simulink model "P2Simulink"  (R2023b)
settings: Solver=VariableStepAuto  StartTime=0.0  StopTime=100  FixedStep=1  RelTol=1e-3
undefined symbols (not defined in the file or in its folder): DiscIntNeverNeededParam, K, kw, LA, R, tau, Ts, x, y
settings Model: PauseTimes=100  Creator=rpl  LastModifiedBy=rpl

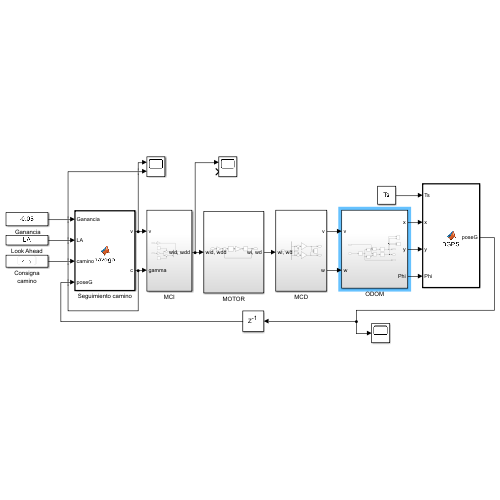
[thumbnail: Simulink's stored preview of the top-level diagram]
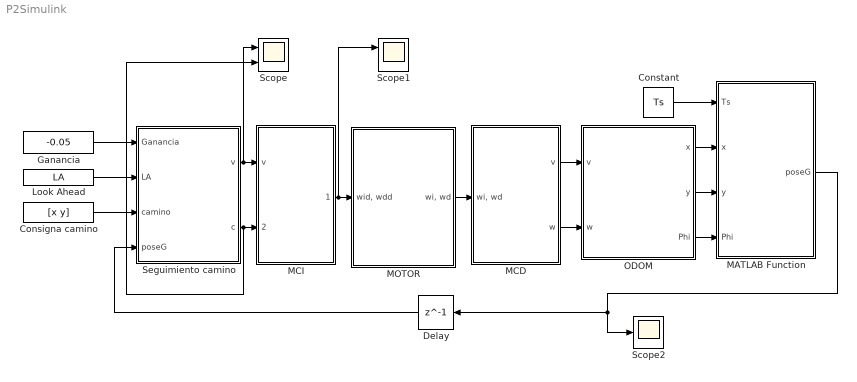
== system P2Simulink ==
  " Ganancia" : Constant  Value=-0.05
  Consigna camino : Constant  Value=[x y]  SampleTime=Ts
  Constant : Constant  Value=Ts
  Delay : Delay  DelayLength=1  InitialCondition=[0; 0; 0]
  Look Ahead : Constant  Value=LA
  MATLAB Function : MATLAB Function  TreatAsAtomicUnit=on
  MCD : Subsystem
  MCI : Subsystem
  MOTOR : Subsystem
  ODOM : Subsystem
  Scope : Scope  NumInputPorts=2
  Scope1 : Scope  NumInputPorts=2
  Scope2 : Scope
  Seguimiento camino : MATLAB Function  TreatAsAtomicUnit=on
  wires:
  MOTOR/1("wi, wd") -> MCD/1("wi, wd")
  Consigna camino/1 -> Seguimiento camino/3(camino)
  MCD/1(v) -> ODOM/1(v)
  MCD/2(w) -> ODOM/2(w)
  MATLAB Function/1(poseG) -> Scope2/1, Delay/1
  MCI/1("wid, wdd") -> Scope1/1, MOTOR/1("wid, wdd")
  Seguimiento camino/1(v) -> Scope/1, MCI/1(v)
  Seguimiento camino/2(c) -> Scope/2, MCI/2(gamma)
  " Ganancia"/1 -> Seguimiento camino/1(Ganancia)
  Constant/1 -> MATLAB Function/1(Ts)
  Look Ahead/1 -> Seguimiento camino/2(LA)
  Delay/1 -> Seguimiento camino/4(poseG)
  ODOM/1(x) -> MATLAB Function/2(x)
  ODOM/2(y) -> MATLAB Function/3(y)
  ODOM/3(Phi) -> MATLAB Function/4(Phi)

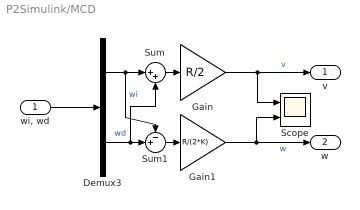
== system P2Simulink/MCD ==
  "wi, wd" : Inport
  Demux3 : Demux  Outputs=2
  Gain : Gain  Gain=R/2
  Gain1 : Gain  Gain=R/(2*K)
  Scope : Scope  NumInputPorts=2
  Sum : Sum  Inputs=|++
  Sum1 : Sum  Inputs=-+|
  v : Outport
  w : Outport  Port=2
  wires:
  Sum/1 -> Gain/1
  Gain/1 -> Scope/1, v/1  "v"
  Demux3/2 -> Sum/2, Sum1/2  "wd"
  Demux3/1 -> Sum1/1, Sum/1  "wi"
  Sum1/1 -> Gain1/1
  Gain1/1 -> Scope/2, w/1  "w"
  "wi, wd"/1 -> Demux3/1

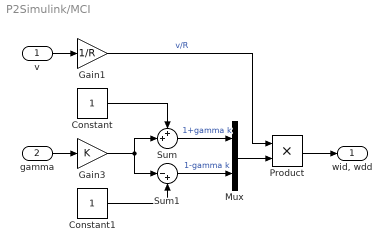
== system P2Simulink/MCI ==
  v : Inport
  gamma : Inport  Port=2
  Constant : Constant
  Constant1 : Constant
  Gain1 : Gain  Gain=1/R
  Gain3 : Gain  Gain=K
  Mux : Mux  Inputs=2
  Product : Product
  Sum : Sum  Inputs=++|
  Sum1 : Sum  Inputs=|-+
  "wid, wdd" : Outport
  wires:
  v/1 -> Gain1/1
  Sum/1 -> Mux/1  "1+gamma k"
  Mux/1 -> Product/2
  Sum1/1 -> Mux/2  "1-gamma k"
  gamma/1 -> Gain3/1
  Gain1/1 -> Product/1  "v/R"
  Product/1 -> "wid, wdd"/1
  Constant/1 -> Sum/1
  Gain3/1 -> Sum1/1, Sum/2
  Constant1/1 -> Sum1/2

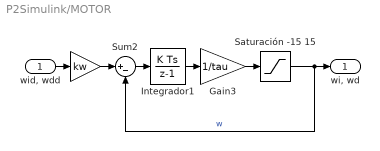
== system P2Simulink/MOTOR ==
  "wid, wdd" : Inport
  " " : Gain  Gain=kw
  Gain3 : Gain  Gain=1/tau
  Integrador1 : DiscreteIntegrator  SampleTime=-1  ICPrevOutput=DiscIntNeverNeededParam  ICPrevScaledInput=DiscIntNeverNeededParam
  Saturación -15 15 : Saturate  UpperLimit=15  LowerLimit=-15
  Sum2 : Sum  Inputs=|+-
  "wi, wd" : Outport
  wires:
  Gain3/1 -> Saturación -15 15/1
  Integrador1/1 -> Gain3/1
  Sum2/1 -> Integrador1/1
  Saturación -15 15/1 -> Sum2/2, "wi, wd"/1  "w"
  "wid, wdd"/1 -> " "/1
  " "/1 -> Sum2/1

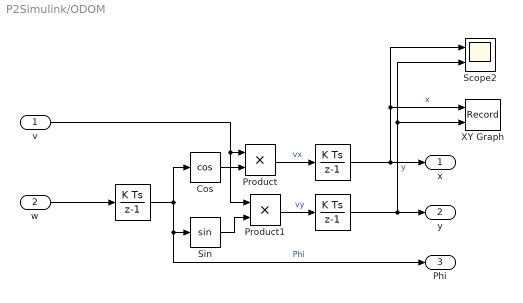
== system P2Simulink/ODOM ==
  v : Inport
  w : Inport  Port=2
  " " : DiscreteIntegrator  SampleTime=-1  ICPrevOutput=DiscIntNeverNeededParam  ICPrevScaledInput=DiscIntNeverNeededParam
  "  " : DiscreteIntegrator  SampleTime=-1  ICPrevOutput=DiscIntNeverNeededParam  ICPrevScaledInput=DiscIntNeverNeededParam
  "   " : DiscreteIntegrator  SampleTime=-1  ICPrevOutput=DiscIntNeverNeededParam  ICPrevScaledInput=DiscIntNeverNeededParam
  Cos : Trigonometry  Operator=cos
  Product : Product
  Product1 : Product
  Scope2 : Scope  NumInputPorts=2
  Sin : Trigonometry
  XY Graph : Record  FileSettingsInternal="{\"entries\":[{\"content\":{\"excelSettings\":{\"content\":{},\"type\":\"Streamout.ExcelSettings\"}},\"type\":\"Streamout.FileSettingStorage\",\"uuid\":\"\"}],\"packageUris\":[\"http:\\/\\/schema.mathworks.com\\/mf0\\/streamout_blocks\\/R2020a\"],\"version\":\"1.0\"}"  Layout=[1 1]  SignalsInternal="{\"entries\":[{\"content\":{\"signals\":[{\"content\":{\"blockPath\":[],\"dimensions\":[1],\"domain\":\"\",\"lineColor\":\"#a2142f\",\"plots\":[ 1 ],\"port\":1,\"sid\":[\"\"],\"signalID\":1,\"signalName\":\"x\"},\"type\":\"RecordBlkView.Signal\",\"uuid\":\"\"},{\"content\":{\"blockPath\":[],\"dimensions\":[1],\"domain\":\"\",\"lineColor\":\"#139fff\",\"plots\":[ 1 ],\"port\":2,\"sid\":[\"\"],\"signalID\":2,\"signalName\":\"y\"},\"type\":\"RecordBlkView.Signal\",\"uuid\":\"\"}]},\"type\":\"RecordBlkView.InputSignals\",\"uuid\":\"\"}],\"packageUris\":[\"http:\\/\\/schema.mathworks.com\\/mf0\\/streamout_blocks\\/R2020a\"],\"version\":\"1.0\"}"  VisualizationBindings="{\"xyplotplugin\":{\"info\":[{\"series\":[{\"bindingParametersList\":[{\"parameter\":\"X-Axis\",\"signalID\":1,\"signalName\":\"x\"},{\"parameter\":\"Y-Axis\",\"signalID\":2,\"signalName\":\"y\"}],\"seriesID\":0}],\"subplotID\":1}]}}"  CompatibilityTag=XY
  x : Outport
  y : Outport  Port=2
  Phi : Outport  Port=3
  wires:
  Cos/1 -> Product/2
  w/1 -> "   "/1
  "   "/1 -> Cos/1, Phi/1, Sin/1  "Phi"
  Product/1 -> "  "/1  "vx"
  Sin/1 -> Product1/2
  "  "/1 -> x/1, Scope2/1, XY Graph/1  "x"
  v/1 -> Product1/1, Product/1
  Product1/1 -> " "/1  "vy"
  " "/1 -> y/1, XY Graph/2, Scope2/2  "y"

== matlab function P2Simulink/Seguimiento camino ==
  data: Ganancia input; LA input; camino input; poseG input; v output; c output
function [v, c]= navega(Ganancia, LA, camino, poseG)
    
    % Comprobar si llegamos al final del camino y parar el robot
    persistent paso;
    if isempty(paso)
        paso = 1;
    end
    if paso >= length(camino)
        c = 0;
        v = 0;
    else
        % Cálculo de distancia hasta siguiente punto del camino
        deltaX = camino(paso, 1) - poseG(1);
        deltaY = camino(paso, 2) - poseG(2);
        
        % Si la distancia es menor que el look ahead, cambiar de paso
        dist = sqrt(deltaX^2 + deltaY^2);
        if (dist < LA)
            paso = paso + 1
        end

        % Calcular la curvatura
        Phi = poseG(3); % orientación del robot
        TRot = [cos(Phi), sin(Phi);-sin(Phi), cos(Phi)];
        xn_hat = TRot * [deltaX; deltaY];
        gamma = atan2(xn_hat(2), xn_hat(1))

        % Devolver las consignas de velocidad y curvatura
        v = 1.2; % Velocidad lineal del motor (metros/segundo)
        c = gamma*Ganancia
    end

== matlab function P2Simulink/MATLAB Function ==
  data: Ts input; x input; poseG output; y input; Phi input
function poseG = DGPS(Ts, x, y, Phi)
    %DGPS Simulacion de un receptor GPS diferencial 
    % PoseO: posicion real en el plano del receptor según la odometría
    % poseG: coordenadas X, Y, Phi medidas por el GPS

    %persistent tSim
    %persistent ultLectura
    %persistent ultPose;
    %% Inicializar el tiempo de simulación y el tiempo de última lectura
    %if isempty(tSim)
    %    tSim = 0;
    %    ultLectura = -1;
    %    ultPose = [0 0 0]';
    %end

    %% Actualizar valores sólo si pasaron 0.3 s desde última lectura
    %T_GPS_RTK = 0.3; % Periodo de medición del GPS diferencial (segundos)
    %tSim = tSim + Ts;
    %if ultLectura < tSim + T_GPS_RTK 
    %    ultLectura = tSim;
        ruido = sqrtm([0.4 -0.014 0; -0.014 0.5 0;0 0 0.1])*randn(3, 1);        
        %!ultPose = [x+ruido(1); y+ruido(2); Phi+ruido(3)];
        ultPose = real([x+ruido(1); y+ruido(2); Phi+ruido(3)]);
    %end
    poseG = ultPose;
end
